simulink library "carnot"  (R2013b)
settings: Solver=ode45  StartTime=0.0  StopTime=10.0  RelTol=1e-3
undefined symbols (not defined in the file or in its folder): A, acol, Ahabit, Awin, Azimuth_Angle, AziWin, B, C, c1, c4, capc, caph, CarnotCallbacks_Density, CarnotCallbacks_Enthalpy, CarnotCallbacks_Enthalpy2Temperature, CarnotCallbacks_Entropy, CarnotCallbacks_Evaporation_Enthalpy, CarnotCallbacks_GlobalMessageLevel, CarnotCallbacks_Grashof, CarnotCallbacks_Heat_Capacity, CarnotCallbacks_Kinematic_Viscosity, CarnotCallbacks_Prandtl, CarnotCallbacks_Saturation_Property, CarnotCallbacks_Saturation_Temperature, CarnotCallbacks_Saturation_Value_Water, CarnotCallbacks_Specific_Volume, CarnotCallbacks_Thermal_Conductivity, CarnotCallbacks_Vapour_Content, CarnotCallbacks_Vapour_Pressure, con, cond, d, Dd, density, dfin, dia, DiameterLastPiece, DPConstant, dpipe, DPLinear, DPQuadratic, emission_out, fluid, FluidMix, FluidType, FPC, frame, g, GeodeticHeight, Gwin, heat_capacity, hgt, HP, Hroom, ID, inlet, K, l, lin, lpipe ... (+29)
undefined symbols (not defined in the file): c2, c3, c5, c6, cwall, dactive, height, mc, mID, rho, tau, UAneighbour, UAwall, uloss
libraries: carnot x333, simulink x25, simulink_extras x7
(part 3 of 16)

== system carnot/Basic/Hydraulics ==
  Flow_Mixer_basic : Subsystem  mask(Flow Mixer Basic){}
      mask help:
      | The flow mixer calculated the temperature and massflow of 2 entering flows.
      | The temperature is calculated in the block Mix_T_Mdot.
      | The flow diversion fdiv (feed back to the flow diverter) takes care that the pressure drop in the 2 branches is the same. The resulting pressure drop coefficients are calulated in the s-function mix_flow (uses solve_quadratic_equation in Carlib).
      mask Help: web(fullfile(path_carnot('help'),'Flow_Mixer_basic.html'),'-helpbrowser')
      mask Display: disp('Flow\nMixer')
  Grashof : Subsystem  LoadFcn=CarnotCallbacks_Grashof('LoadFcn');  VariantControl=CarlibClassic  mask(Grashof){DEBUGLEVEL=WARNINGLEVEL, MAXTOTALMESSAGES=inf, MAXCONSECUTIVEMESSAGES=inf, WRITETOFILE=0, FILENAME='errors.txt'}
      mask prompts: DEBUGLEVEL "Debug level"; MAXTOTALMESSAGES "maximum number of total warning"; MAXCONSECUTIVEMESSAGES "maximum number of consecutive warnings"; WRITETOFILE "write messages to file"; FILENAME "filename for error messages"
      mask help:
      | Calculates the Gashof number. You may use the block "GlobalMessageLevel" in the Toolbox to handle the debugging messages.
      | Inputs are:
      | 1   wall temperature - scalar or vector
      | 2   temperature at infinite distance - scalar
      | 3   pressure - scalar
      | 4   fluid type (see below) - scalar
      | 5   fluid_mix - scalar
      | 6   characteristic dimension - scalar
      |
      | FluidType        Remarks
      | 1: water          fluid mix is vapourcontent in the 2-phase region
      | 2: air              fluid mix is (kg water) / (kg dry air)
      | 3: cotton oil       -
      | 4: silicone oil     -
      | 5: water-glycol   fluid mix is volume partition [0..1] of propylen glycol
      | 6: Tyfocor LS     function only available in liquid phase
      | 7: Water Constant = 998.21 kg/m³ (water at 20°C)
      | 8: Air Constant   = 1.118 kg/m³ (air at 20°C)
      mask init:
      | %global debug level
      | [DEBUGLEVEL, MAXTOTALMESSAGES, MAXCONSECUTIVEMESSAGES, WRITETOFILE, FILENAME] = CarnotCallbacks_Grashof('CheckDebugLevels', DEBUGLEVEL, MAXTOTALMESSAGES, MAXCONSECUTIVEMESSAGES, WRITETOFILE, FILENAME);
      mask Help: web(fullfile(path_carnot('help'),'Grashof.html'),'-helpbrowser')
      mask TypeOptions DEBUGLEVEL: DEBUGLEVEL | INFOLEVEL | WARNINGLEVEL | ERRORLEVEL | FATALLEVEL | NOLEVEL
      mask DialogControl ParameterTabVar0 Prompt: Debugging
  Mix_T_Mdot : Subsystem  mask(mix_temperature){mixcalc=Tmix = (mdot1*T1 + mdot2*T2)/(mdot1+mdot2)}
      mask prompts: mixcalc "Calculation of mixture :"
      mask help:
      | Calculate the temperature of the mixture of two flows. Uses enthalpy balance for humid air. Liquids may be mixed by the (faster and approximate) equation:
      | Tmix = (mdot1*T1 + mdot2*T2)/(mdot1+mdot2)
      mask Help: web(fullfile(path_carnot('help'),'Mix_T_Mdot.html'),'-helpbrowser')
      mask TypeOptions mixcalc: Tmix = (mdot1*T1 + mdot2*T2)/(mdot1+mdot2) | Enthalpy balance
  Prandtl : Subsystem  LoadFcn=CarnotCallbacks_Prandtl('LoadFcn');  InitFcn=load('THB.mat');  VariantControl=CarlibClassic  mask(Prandtl){INPUTARGUMENTS=state variables (classic), DEBUGLEVEL=WARNINGLEVEL, MAXTOTALMESSAGES=inf, MAXCONSECUTIVEMESSAGES=inf, WRITETOFILE=0, FILENAME='errors.txt'}
      mask prompts: INPUTARGUMENTS "Input arguments"; DEBUGLEVEL "Debug level"; MAXTOTALMESSAGES "maximum number of total warning"; MAXCONSECUTIVEMESSAGES "maximum number of consecutive warnings"; WRITETOFILE "write messages to file"; FILENAME "filename for error messages"
      mask help:
      | Calculates the Prandtl number for given materials properties.
      | You may use the block "GlobalMessageLevel" in the Toolbox to handle the debugging messages.
      | FluidType        Remarks
      | 1: water          fluid mix is vapourcontent in the 2-phase region
      | 2: air              fluid mix is (kg water) / (kg dry air)
      | 3: cotton oil       -
      | 4: silicone oil     -
      | 5: water-glycol   fluid mix is volume partition [0..1] of propylen glycol
      | 6: Tyfocor LS     function only available in liquid phase
      | 7: Water Constant = 998.21 kg/m³ (water at 20°C)
      | 8: Air Constant   = 1.118 kg/m³ (air at 20°C)
      mask init:
      | %Inports
      | CarnotCallbacks_Prandtl('CreateInports');
      | 
      | %global debug level
      | [DEBUGLEVEL, MAXTOTALMESSAGES, MAXCONSECUTIVEMESSAGES, WRITETOFILE, FILENAME] = CarnotCallbacks_Prandtl('CheckDebugLevels', DEBUGLEVEL, MAXTOTALMESSAGES, MAXCONSECUTIVEMESSAGES, WRITETOFILE, FILENAME);
      mask Help: web(fullfile(path_carnot('help'),'Prandtl.html'),'-helpbrowser')
      mask TypeOptions INPUTARGUMENTS: state variables (classic) | THB | THV
      mask Callback INPUTARGUMENTS: CarnotCallbacks_Prandtl('MaskVisibilities');
      mask TypeOptions DEBUGLEVEL: DEBUGLEVEL | INFOLEVEL | WARNINGLEVEL | ERRORLEVEL | FATALLEVEL | NOLEVEL
  Pump_basic : Subsystem  mask(basic Pump){mdotmax=1200/3600, fluid_id=1, mix=0, dia=0.02, power=30, p0=3e5, hgt=0, ID=ID}
      mask prompts: mdotmax "massflow rate [kg/s]"; fluid_id "fluid"; mix "percentage of fluid mix [0..1]"; dia "diameter at in- and outlet [m]"; power "electric power consumption [W]"; p0 "system pressure [Pa]"; hgt "static height in m (positive value above ground)"; ID "ID (pressure drop calculation mode)"
      mask help:
      | Set constant massflow rate according to the control signal.
      | The pump is a very basic model, sometimes creating algebraic loops. If you have problems with algebraic loops, use "Pump_const" instead.
      | ID for pressure drop calculation:
      |     1    .. 9999 No Pressure Drop
      |     10001..19999 Pressure Drop from Massflow
      |     20001..inf   Full Pressure Drop with Static Height
      mask init:
      | mix = min(1, max(0, mix));
      | dia = max(0.001, dia);
      mask Help: web(fullfile(path_carnot('help'),'Pump_basic.html'),'-helpbrowser')
      mask Display: plot(0,0,100,100,[40,70,40,30,30,40,60,70,70,60,40],[70,50,30,40,60,70,70,60,40,30,30])
  Reynolds : Subsystem  mask(Reynolds number){}
      mask help:
      | Calculates the Reynolds number for a flow, give the characteristic dimension as an input.
      | Pipe: diameter
      | Duct: 4 * cross_section / perimeter
      | Plate: length
      mask Help: web(fullfile(path_carnot('help'),'Reynolds.html'),'-helpbrowser')
  THBCreator : Subsystem  InitFcn=load('THB.mat');  mask(THBCreator){Inport_ID=on, Inport_T=on, Inport_mdot=on, Inport_p=on, Inport_type=on, Inport_mix=on, Inport_d=on, Inport_c=on, Inport_l=on, Inport_q=on, Inport_LH=on, Inport_H=on, ID=20001, T=20, mdot=0, p=1e5, FluidType=1, FluidMix=0, d=0.01, c=0, l=0, q=0, LH=0, H=0, Annotation_ID=off, Annotation_T=off, Annotation_mdot=off, Annotation_p=off, Annotation_type=off, Annotation_mix=off, Annotation_d=off, Annotation_c=off, Annotation_l=off, Annotation_q=off, Annotation_LH=off, Annotation_H=off}
      mask prompts: Inport_ID "ID as inport"; Inport_T "temperature as inport"; Inport_mdot "mass flow rate as inport"; Inport_p "pressure as inport"; Inport_type "fluid type as inport"; Inport_mix "fluid mix as inport"; Inport_d "diameter last piece as inport"; Inport_c "constant pressure drop coefficient as inport"; Inport_l "linear pressure drop coefficient as inport"; Inport_q "quadratic pressure drop coefficient as inport"; Inport_LH "hydraulic inductance as inport"; Inport_H "geodetic height as inport"; ID "ID [1]"; T "temperature [°C]"; mdot "mass flow rate [kg/s]"; p "pressure [Pa]"; FluidType "fluid type [enum]"; FluidMix "fluid mix [1]"; d "diameter last piece [m]"; c "constant pressure drop coefficient [Pa]"; l "linear pressure drop coefficient [Pa/(kg/s)]"; q "quadratic pressure drop coefficient [Pa/(kg/s)²]"; LH "hydraulic inductance [1/m]"; H "geodetic height"; Annotation_ID "ID as annotation"; Annotation_T "temperature as annotation"; Annotation_mdot "mass flow rate as annotation"; Annotation_p "pressure as annotation"; Annotation_type "fluid type as annotation"; Annotation_mix "fluid mix as annotation"; Annotation_d "diameter last piece as annotation"; Annotation_c "constant pressure drop coefficient as annotation"; Annotation_l "linear pressure drop coefficient as annotation"; Annotation_q "quadratic pressure drop coefficient as annotation"; Annotation_LH "hydraulic inductance as annotation"; Annotation_H "geodetic height as annotation"
      mask help: This block creates a THB from input signals.
      mask init:
      | MaskValue = get_param(gcb,'MaskValues');
      |     
      | if strcmp(MaskValue{1},'on') %ID
      |     if ~strcmp(get_param([gcb,'/ID'],'BlockType'),'Inport')
      |         delete_line(gcb,'ID/1','BusCreator/1'); %delete connection
      |         delete_block([gcb,'/ID']); %delete block
      |         add_block('built-in/Inport',[gcb,'/ID']); %add new block
      |         set_param([gcb, '/ID'],'Position',[50   1*50+8   50+30   1*50+8+14]); %set new block's position
      |         add_line(gcb,'ID/1','BusCreator/1'); %add new connection
      |         handles=get_param([gcb, '/ID'],'LineHandles'); %get line handles
      |         set(handles.Outport(1),'Name','ID'); %set line name
      |     end
      | else
      |     if ~strcmp(get_param([gcb,'/ID'],'BlockType'),'Constant')
      |         delete_line(gcb,'ID/1','BusCreator/1'); %delete connection
      |         delete_block([gcb,'/ID']); %delete block
      |         add_block('built-in/Constant',[gcb,'/ID']); %add new block
      |         set_param([gcb, '/ID'],'Position',[50   1*50   50+30   1*50+30]); %set new block's position
      |         set_param([gcb, '/ID'],'Value','ID'); %set mask varible as value
      |         add_line(gcb,'ID/1','BusCreator/1'); %add new connection
      |         handles=get_param([gcb, '/ID'],'LineHandles'); %get line handles
      |         set(handles.Outport(1),'Name','ID'); %set line name
      |     end
      | end
      | 
      | if strcmp(MaskValue{2},'on') %T
      |     if ~strcmp(get_param([gcb,'/Temperature'],'BlockType'),'Inport')
      |         delete_line(gcb,'Temperature/1','BusCreator/2'); %delete connection
      |         delete_block([gcb,'/Temperature']); %delete block
      |         add_block('built-in/Inport',[gcb,'/Temperature']); %add new block
      |         set_param([gcb, '/Temperature'],'Position',[50   2*50+8   50+30   2*50+8+14]); %set new block's position
      |         add_line(gcb,'Temperature/1','BusCreator/2'); %add new connection
      |         handles=get_param([gcb, '/Temperature'],'LineHandles'); %get line handles
      |         set(handles.Outport(1),'Name','Temperature'); %set line name
      |     end
      | else
      |     if ~strcmp(get_param([gcb,'/Temperature'],'BlockType'),'Constant')
      |         delete_line(gcb,'Temperature/1','BusCreator/2'); %delete connection
      |         delete_block([gcb,'/Temperature']); %delete block
      |         add_block('built-in/Constant',[gcb,'/Temperature']); %add new block
      |         set_param([gcb, '/Temperature'],'Position',[50   2*50   50+30   2*50+30]); %set new block's position
      |         set_param([gcb, '/Temperature'],'Value','T'); %set mask varible as value
      |         add_line(gcb,'Temperature/1','BusCreator/2'); %add new connection
      |         handles=get_param([gcb, '/Temperature'],'LineHandles'); %get line handles
      |         set(handles.Outport(1),'Name','Temperature'); %set line name
      |     end
      | end
      | 
      | if strcmp(MaskValue{3},'on') %MassFlow
      |     if ~strcmp(get_param([gcb,'/MassFlow'],'BlockType'),'Inport')
      |         delete_line(gcb,'MassFlow/1','BusCreator/3'); %delete connection
      |         delete_block([gcb,'/MassFlow']); %delete block
      |         add_block('built-in/Inport',[gcb,'/MassFlow']); %add new block
      |         set_param([gcb, '/MassFlow'],'Position',[50   3*50+8   50+30   3*50+8+14]); %set new block's position
      |         add_line(gcb,'MassFlow/1','BusCreator/3'); %add new connection
      |         handles=get_param([gcb, '/MassFlow'],'LineHandles'); %get line handles
      |         set(handles.Outport(1),'Name','MassFlow'); %set line name
      |     end
      | else
      |     if ~strcmp(get_param([gcb,'/MassFlow'],'BlockType'),'Constant')
      |         delete_line(gcb,'MassFlow/1','BusCreator/3'); %delete connection
      |         delete_block([gcb,'/MassFlow']); %delete block
      |         add_block('built-in/Constant',[gcb,'/MassFlow']); %add new block
      |         set_param([gcb, '/MassFlow'],'Position',[50   3*50   50+30   3*50+30]); %set new block's position
      |         set_param([gcb, '/MassFlow'],'Value','mdot'); %set mask varible as value
      |         add_line(gcb,'MassFlow/1','BusCreator/3'); %add new connection
      |         handles=get_param([gcb, '/MassFlow'],'LineHandles'); %get line handles
      |         set(handles.Outport(1),'Name','MassFlow'); %set line name
      |     end
      | end
      | 
      | if strcmp(MaskValue{4},'on') %Pressure
      |     if ~strcmp(get_param([gcb,'/Pressure'],'BlockType'),'Inport')
      |         delete_line(gcb,'Pressure/1','BusCreator/4'); %delete connection
      |         delete_block([gcb,'/Pressure']); %delete block
      |         add_block('built-in/Inport',[gcb,'/Pressure']); %add new block
      |         set_param([gcb, '/Pressure'],'Position',[50   4*50+8   50+30   4*50+8+14]); %set new block's position
      |         add_line(gcb,'Pressure/1','BusCreator/4'); %add new connection
      |         handles=get_param([gcb, '/Pressure'],'LineHandles'); %get line handles
      |         set(handles.Outport(1),'Name','Pressure'); %set line name
      |     end
      | else
      |     if ~strcmp(get_param([gcb,'/Pressure'],'BlockType'),'Constant')
      |         delete_line(gcb,'Pressure/1','BusCreator/4'); %delete connection
      |         delete_block([gcb,'/Pressure']); %delete block
      |         add_block('built-in/Constant',[gcb,'/Pressure']); %add new block
      |         set_param([gcb, '/Pressure'],'Position',[50   4*50   50+30   4*50+30]); %set new block's position
      |         set_param([gcb, '/Pressure'],'Value','p'); %set mask varible as value
      |         add_line(gcb,'Pressure/1','BusCreator/4'); %add new connection
      |         handles=get_param([gcb, '/Pressure'],'LineHandles'); %get line handles
      |         set(handles.Outport(1),'Name','Pressure'); %set line name
      |     end
      | end
      | 
      | if strcmp(MaskValue{5},'on') %FluidType
      |     if ~strcmp(get_param([gcb,'/FluidType'],'BlockType'),'Inport')
      |         delete_line(gcb,'FluidType/1','BusCreator/5'); %delete connection
      |         delete_block([gcb,'/FluidType']); %delete block
      |         add_block('built-in/Inport',[gcb,'/FluidType']); %add new block
      |         set_param([gcb, '/FluidType'],'Position',[50   5*50+8   50+30   5*50+8+14]); %set new block's position
      |         add_line(gcb,'FluidType/1','BusCreator/5'); %add new connection
      |         handles=get_param([gcb, '/FluidType'],'LineHandles'); %get line handles
      |         set(handles.Outport(1),'Name','FluidType'); %set line name
      |     end
      | else
      |     if ~strcmp(get_param([gcb,'/FluidType'],'BlockType'),'Constant')
      |         delete_line(gcb,'FluidType/1','BusCreator/5'); %delete connection
      |         delete_block([gcb,'/FluidType']); %delete block
      |         add_block('built-in/Constant',[gcb,'/FluidType']); %add new block
      |         set_param([gcb, '/FluidType'],'Position',[50   5*50   50+30   5*50+30]); %set new block's position
      |         set_param([gcb, '/FluidType'],'Value','FluidType'); %set mask varible as value
      |         add_line(gcb,'FluidType/1','BusCreator/5'); %add new connection
      |         handles=get_param([gcb, '/FluidType'],'LineHandles'); %get line handles
      |         set(handles.Outport(1),'Name','FluidType'); %set line name
      |     end
      | end
      | 
      | if strcmp(MaskValue{6},'on') %FluidMix
      |     if ~strcmp(get_param([gcb,'/FluidMix'],'BlockType'),'Inport')
      |         delete_line(gcb,'FluidMix/1','BusCreator/6'); %delete connection
      |         delete_block([gcb,'/FluidMix']); %delete block
      |         add_block('built-in/Inport',[gcb,'/FluidMix']); %add new block
      |         set_param([gcb, '/FluidMix'],'Position',[50   6*50+8   50+30   6*50+8+14]); %set new block's position
      |         add_line(gcb,'FluidMix/1','BusCreator/6'); %add new connection
      |         handles=get_param([gcb, '/FluidMix'],'LineHandles'); %get line handles
      |         set(handles.Outport(1),'Name','FluidMix'); %set line name
      |     end
      | else
      |     if ~strcmp(get_param([gcb,'/FluidMix'],'BlockType'),'Constant')
      |         delete_line(gcb,'FluidMix/1','BusCreator/6'); %delete connection
      |         delete_block([gcb,'/FluidMix']); %delete block
      |         add_block('built-in/Constant',[gcb,'/FluidMix']); %add new block
      |         set_param([gcb, '/FluidMix'],'Position',[50   6*50   50+30   6*50+30]); %set new block's position
      |         set_param([gcb, '/FluidMix'],'Value','FluidMix'); %set mask varible as value
      |         add_line(gcb,'FluidMix/1','BusCreator/6'); %add new connection
      |         handles=get_param([gcb, '/FluidMix'],'LineHandles'); %get line handles
      |         set(handles.Outport(1),'Name','FluidMix'); %set line name
      |     end
      | end
      | 
      | if strcmp(MaskValue{7},'on') %DiameterLastPiece
      |     if ~strcmp(get_param([gcb,'/DiameterLastPiece'],'BlockType'),'Inport')
      |         delete_line(gcb,'DiameterLastPiece/1','BusCreator/7'); %delete connection
      |         delete_block([gcb,'/DiameterLastPiece']); %delete block
      |         add_block('built-in/Inport',[gcb,'/DiameterLastPiece']); %add new block
      |         set_param([gcb, '/DiameterLastPiece'],'Position',[50   7*50+8   50+30   7*50+8+14]); %set new block's position
      |         add_line(gcb,'DiameterLastPiece/1','BusCreator/7'); %add new connection
      |         handles=get_param([gcb, '/DiameterLastPiece'],'LineHandles'); %get line handles
      |         set(handles.Outport(1),'Name','DiameterLastPiece'); %set line name
      |     end
      | else
      |     if ~strcmp(get_param([gcb,'/DiameterLastPiece'],'BlockType'),'Constant')
      |         delete_line(gcb,'DiameterLastPiece/1','BusCreator/7'); %delete connection
      |         delete_block([gcb,'/DiameterLastPiece']); %delete block
      |         add_block('built-in/Constant',[gcb,'/DiameterLastPiece']); %add new block
      |         set_param([gcb, '/DiameterLastPiece'],'Position',[50   7*50   50+30   7*50+30]); %set new block's position
      |         set_param([gcb, '/DiameterLastPiece'],'Value','d'); %set mask varible as value
      |         add_line(gcb,'DiameterLastPiece/1','BusCreator/7'); %add new connection
      |         handles=get_param([gcb, '/DiameterLastPiece'],'LineHandles'); %get line handles
      |         set(handles.Outport(1),'Name','DiameterLastPiece'); %set line name
      |     end
      | end
      | 
      | if strcmp(MaskValue{8},'on') %DPConstant
      |     if ~strcmp(get_param([gcb,'/DPConstant'],'BlockType'),'Inport')
      |         delete_line(gcb,'DPConstant/1','BusCreator/8'); %delete connection
      |         delete_block([gcb,'/DPConstant']); %delete block
      |         add_block('built-in/Inport',[gcb,'/DPConstant']); %add new block
      |         set_param([gcb, '/DPConstant'],'Position',[50   8*50+8   50+30   8*50+8+14]); %set new block's position
      |         add_line(gcb,'DPConstant/1','BusCreator/8'); %add new connection
      |         handles=get_param([gcb, '/DPConstant'],'LineHandles'); %get line handles
      |         set(handles.Outport(1),'Name','DPConstant'); %set line name
      |     end
      | else
      |     if ~strcmp(get_param([gcb,'/DPConstant'],'BlockType'),'Constant')
      |         delete_line(gcb,'DPConstant/1','BusCreator/8'); %delete connection
      |         delete_block([gcb,'/DPConstant']); %delete block
      |         add_block('built-in/Constant',[gcb,'/DPConstant']); %add new block
      |         set_param([gcb, '/DPConstant'],'Position',[50   8*50   50+30   8*50+30]); %set new block's position
      |         set_param([gcb, '/DPConstant'],'Value','c'); %set mask varible as value
      |         add_line(gcb,'DPConstant/1','BusCreator/8'); %add new connection
      |         handles=get_param([gcb, '/DPConstant'],'LineHandles'); %get line handles
      |         set(handles.Outport(1),'Name','DPConstant'); %set line name
      |     end
      | end
      | 
      | if strcmp(MaskValue{9},'on') %DPLinear
      |     if ~strcmp(get_param([gcb,'/DPLinear'],'BlockType'),'Inport')
      |         delete_line(gcb,'DPLinear/1','BusCreator/9'); %delete connection
      |         delete_block([gcb,'/DPLinear']); %delete block
      |         add_block('built-in/Inport',[gcb,'/DPLinear']); %add new block
      |         set_param([gcb, '/DPLinear'],'Position',[50   9*50+8   50+30   9*50+8+14]); %set new block's position
      |         add_line(gcb,'DPLinear/1','BusCreator/9'); %add new connection
      |         handles=get_param([gcb, '/DPLinear'],'LineHandles'); %get line handles
      |         set(handles.Outport(1),'Name','DPLinear'); %set line name
      |     end
      | else
      |     if ~strcmp(get_param([gcb,'/DPLinear'],'BlockType'),'Constant')
      |         delete_line(gcb,'DPLinear/1','BusCreator/9'); %delete connection
      |         delete_block([gcb,'/DPLinear']); %delete block
      |         add_block('built-in/Constant',[gcb,'/DPLinear']); %add new block
      |         set_param([gcb, '/DPLinear'],'Position',[50   9*50   50+30   9*50+30]); %set new block's position
      |         set_param([gcb, '/DPLinear'],'Value','l'); %set mask varible as value
      |         add_line(gcb,'DPLinear/1','BusCreator/9'); %add new connection
      |         handles=get_param([gcb, '/DPLinear'],'LineHandles'); %get line handles
      |         set(handles.Outport(1),'Name','DPLinear'); %set line name
      |     end
      | end
      | 
      | if strcmp(MaskValue{10},'on') %DPQuadratic
      |     if ~strcmp(get_param([gcb,'/DPQuadratic'],'BlockType'),'Inport')
      |         delete_line(gcb,'DPQuadratic/1','BusCreator/10'); %delete connection
      |         delete_block([gcb,'/DPQuadratic']); %delete block
      |         add_block('built-in/Inport',[gcb,'/DPQuadratic']); %add new block
      |         set_param([gcb, '/DPQuadratic'],'Position',[50   10*50+8   50+30   10*50+8+14]); %set new block's position
      |         add_line(gcb,'DPQuadratic/1','BusCreator/10'); %add new connection
      |         handles=get_param([gcb, '/DPQuadratic'],'LineHandles'); %get line handles
      |         set(handles.Outport(1),'Name','DPQuadratic'); %set line name
      |     end
      | else
      |     if ~strcmp(get_param([gcb,'/DPQuadratic'],'BlockType'),'Constant')
      |         delete_line(gcb,'DPQuadratic/1','BusCreator/10'); %delete connection
      |         delete_block([gcb,'/DPQuadratic']); %delete block
      |         add_block('built-in/Constant',[gcb,'/DPQuadratic']); %add new block
      |         set_param([gcb, '/DPQuadratic'],'Position',[50   10*50   50+30   10*50+30]); %set new block's position
      |         set_param([gcb, '/DPQuadratic'],'Value','q'); %set mask varible as value
      |         add_line(gcb,'DPQuadratic/1','BusCreator/10'); %add new connection
      |         handles=get_param([gcb, '/DPQuadratic'],'LineHandles'); %get line handles
      |         set(handles.Outport(1),'Name','DPQuadratic'); %set line name
      |     end
      | end
      | 
      | if strcmp(MaskValue{11},'on') %HydraulicInductance
      |     if ~strcmp(get_param([gcb,'/HydraulicInductance'],'BlockType'),'Inport')
      |         delete_line(gcb,'HydraulicInductance/1','BusCreator/11'); %delete connection
      |         delete_block([gcb,'/HydraulicInductance']); %delete block
      |         add_block('built-in/Inport',[gcb,'/HydraulicInductance']); %add new block
      |         set_param([gcb, '/HydraulicInductance'],'Position',[50   11*50+8   50+30   11*50+8+14]); %set new block's position
      |         add_line(gcb,'HydraulicInductance/1','BusCreator/11'); %add new connection
      |         handles=get_param([gcb, '/HydraulicInductance'],'LineHandles'); %get line handles
      |         set(handles.Outport(1),'Name','HydraulicInductance'); %set line name
      |     end
      | else
      |     if ~strcmp(get_param([gcb,'/HydraulicInductance'],'BlockType'),'Constant')
      |         delete_line(gcb,'HydraulicInductance/1','BusCreator/11'); %delete connection
      |         delete_block([gcb,'/HydraulicInductance']); %delete block
      |         add_block('built-in/Constant',[gcb,'/HydraulicInductance']); %add new block
      |         set_param([gcb, '/HydraulicInductance'],'Position',[50   11*50   50+30   11*50+30]); %set new block's position
      |         set_param([gcb, '/HydraulicInductance'],'Value','LH'); %set mask varible as value
      |         add_line(gcb,'HydraulicInductance/1','BusCreator/11'); %add new connection
      |         handles=get_param([gcb, '/HydraulicInductance'],'LineHandles'); %get line handles
      |         set(handles.Outport(1),'Name','HydraulicInductance'); %set line name
      |     end
      | end
      | 
      | if strcmp(MaskValue{12},'on') %GeodeticHeight
      |     if ~strcmp(get_param([gcb,'/GeodeticHeight'],'BlockType'),'Inport')
      |         delete_line(gcb,'GeodeticHeight/1','BusCreator/12'); %delete connection
      |         delete_block([gcb,'/GeodeticHeight']); %delete block
      |         add_block('built-in/Inport',[gcb,'/GeodeticHeight']); %add new block
      |         set_param([gcb, '/GeodeticHeight'],'Position',[50   12*50+8   50+30   12*50+8+14]); %set new block's position
      |         add_line(gcb,'GeodeticHeight/1','BusCreator/12'); %add new connection
      |         handles=get_param([gcb, '/GeodeticHeight'],'LineHandles'); %get line handles
      |         set(handles.Outport(1),'Name','GeodeticHeight'); %set line name
      |     end
      | else
      |     if ~strcmp(get_param([gcb,'/GeodeticHeight'],'BlockType'),'Constant')
      |         delete_line(gcb,'GeodeticHeight/1','BusCreator/12'); %delete connection
      |         delete_block([gcb,'/GeodeticHeight']); %delete block
      |         add_block('built-in/Constant',[gcb,'/GeodeticHeight']); %add new block
      |         set_param([gcb, '/GeodeticHeight'],'Position',[50   12*50   50+30   12*50+30]); %set new block's position
      |         set_param([gcb, '/GeodeticHeight'],'Value','H'); %set mask varible as value
      |         add_line(gcb,'GeodeticHeight/1','BusCreator/12'); %add new connection
      |         handles=get_param([gcb, '/GeodeticHeight'],'LineHandles'); %get line handles
      |         set(handles.Outport(1),'Name','GeodeticHeight'); %set line name
      |     end
      | end
      mask Help:
      | web('THBCreator.html','-helpbrowser'
      | web(fullfile(path_carnot('help'),'THBCreator.html'),'-helpbrowser')
      mask Callback Inport_ID: THBCreator_ParamCallback;
      mask Callback Inport_T: THBCreator_ParamCallback;
      mask Callback Inport_mdot: THBCreator_ParamCallback;
      mask Callback Inport_p: THBCreator_ParamCallback;
      mask Callback Inport_type: THBCreator_ParamCallback;
      mask Callback Inport_mix: THBCreator_ParamCallback;
      mask Callback Inport_d: THBCreator_ParamCallback;
      mask Callback Inport_c: THBCreator_ParamCallback;
      mask Callback Inport_l: THBCreator_ParamCallback;
      mask Callback Inport_q: THBCreator_ParamCallback;
      mask Callback Inport_LH: THBCreator_ParamCallback;
      mask Callback Inport_H: THBCreator_ParamCallback;
      mask Callback Annotation_ID: THBCreator_ParamCallback;
      mask Callback Annotation_T: THBCreator_ParamCallback;
      mask Callback Annotation_mdot: THBCreator_ParamCallback;
      mask Callback Annotation_p: THBCreator_ParamCallback;
      mask Callback Annotation_type: THBCreator_ParamCallback;
      mask Callback Annotation_mix: THBCreator_ParamCallback;
      mask Callback Annotation_d: THBCreator_ParamCallback;
      mask Callback Annotation_c: THBCreator_ParamCallback;
      mask Callback Annotation_l: THBCreator_ParamCallback;
      mask Callback Annotation_q: THBCreator_ParamCallback;
      mask Callback Annotation_LH: THBCreator_ParamCallback;
      mask Callback Annotation_H: THBCreator_ParamCallback;
  Velocity : Subsystem  mask(velocity){}
      mask help: Calculates the velocity in a pipe [m/s] assuming a round pipe. The diameter is taken from the THV-vector.
      mask Help: web(fullfile(path_carnot('help'),'Velocity.html'),'-helpbrowser')
  basic_THB : Subsystem  mask(constant THV){t=t, mdot=mdot, p=p, ID=ID, fluid=fluid, mix=mix, dia=dia, hgt=hgt}
      mask prompts: t "temperature [degree centigrade]"; mdot "massflow [kg/s]"; p "pressure [Pa]"; ID "Caclulation mode"; mix "fluid mixture [0..1]"; dia "diameter [m]"; hgt "Static height in m"
      mask help:
      | Create a constant Thermo-Hydraulic-Vector.
      | Calculation mode:
      |     1 ..  9999 no pressure drop (dp)
      | 10001 .. 19999 dp caused by flowrate
      | 20001 .. inf   dp by flowrate and static height
      mask init:
      | mix = min(1, max(0, mix));
      | dia = max(dia, 0.001);
      | ID = max(ID,1);
      mask Help: web(fullfile(path_carnot('help'),'basic_THB.html'),'-helpbrowser')
  basic_create_THB : Subsystem  mask(create THV){p=p, fluid=fluid, mix=mix, dia=dia, hgt=0, mID=mID}
      mask prompts: p "pressure [Pa]"; mix "fluid mixture [0..1]"; dia "diameter [m]"; hgt "Geodetic height in m"; mID "Calculation mode"
      mask help:
      | Create a THB with the variable input T and mdot. The other value can be set as constants in the mask.
      | Calculation mode:
      |     1 ..  9999 no pressure drop (dp)
      | 10001 .. 19999 dp caused by flowrate
      | 20001 .. inf   dp by flowrate and static height
      mask init:
      | mix = min(1, max(0, mix));
      | dia = max(dia, 0.001);
      mask Help: web(fullfile(path_carnot('help'),'basic_create_THB.html'),'-helpbrowser')
